simulink model "mrefrobotarm_modified_previous_y_previous_u_previous_ref_cover"  (R2018b)
settings: Solver=FixedStepAuto  StartTime=0.0  StopTime=20  RelTol=1e-3  AbsTol=1e-6
undefined symbols (not defined in the file or in its folder): cc, options
libraries: neural x396, simulink x1
(part 5 of 15)

== system mrefrobotarm_modified_previous_y_previous_u_previous_ref_cover/Feed-Forward Neural Network1/Layer 3/Delays 1 ==
  "p{3}" : Inport  PortDimensions=30
      mask Display: e = 0.06;c1 = [120 230 180]/255;c2 = ([120 230 180]+0)/(256+128);c3 = ([120 230 180]+128)/(256+128);patch([0 1 1 0],[0 0 1 1],c1);patch([0 1 1 1-e 1-e 0+e],[0 0 1 1-e 0+e 0+e],c2);patch([0 0 1 1-e 0+e 0+e],[0 1 1 1-e 1-e 0+e],c3);plot([0 1 1 0 0],[0 0 1 1 0]);
  mux : Mux  Inputs=1
      mask Display: e = 0.06;c1 = [120 150 230]/255;c2 = ([120 150 230]+0)/383;c3 = ([120 150 230]+128)/383;patch([0 1 1 0],[0 0 1 1],c1);patch([0 1 1 1-e 1-e 0+e],[0 0 1 1-e 0+e 0+e],c2);patch([0 0 1 1-e 0+e 0+e],[0 1 1 1-e 1-e 0+e],c3);plot([0 1 1 0 0],[0 0 1 1 0]);disp('Mux')
  "pd{3,2}" : Outport
      mask Display: e = 0.06;c1 = [120 230 180]/255;c2 = ([120 230 180]+0)/(256+128);c3 = ([120 230 180]+128)/(256+128);patch([0 1 1 0],[0 0 1 1],c1);patch([0 1 1 1-e 1-e 0+e],[0 0 1 1-e 0+e 0+e],c2);patch([0 0 1 1-e 0+e 0+e],[0 1 1 1-e 1-e 0+e],c3);plot([0 1 1 0 0],[0 0 1 1 0]);
  wires:
  "p{3}"/1 -> mux/1
  mux/1 -> "pd{3,2}"/1

== system mrefrobotarm_modified_previous_y_previous_u_previous_ref_cover/Feed-Forward Neural Network1/Layer 3/LW{3,2} ==
  "ad{3,2}" : Inport  PortDimensions=30
      mask Display: e = 0.06;c1 = [120 230 180]/255;c2 = ([120 230 180]+0)/(256+128);c3 = ([120 230 180]+128)/(256+128);patch([0 1 1 0],[0 0 1 1],c1);patch([0 1 1 1-e 1-e 0+e],[0 0 1 1-e 0+e 0+e],c2);patch([0 0 1 1-e 0+e 0+e],[0 1 1 1-e 1-e 0+e],c3);plot([0 1 1 0 0],[0 0 1 1 0]);
  "IW{3,2}(1,:)'" : Constant  Value=[0.245566465926212396109207247718586586415767669677734375;-0.56322081322037842454619749332778155803680419921875;-0.28991010367060410235495737651945091784000396728515625;0.3869683333504421174353637979947961866855621337890625;0.496517765752567064030387200546101666986942291259765625;-0.320943780837954883988771825897856615483760833740234375;0.0286370319336148211608605862465992686338722705841064453125;-0.15395906619913668489374458658858202397823333740234375;0.51493301451079076525019218024681322276592254638671875;-0.026941881639260277514491548345176852308213710784912109375;-0.05589778476223307424053388103857287205755710601806640625;0.1600136141061642980343293629630352370440959930419921875;-0.2212967731759021561277478440388222225010395050048828125;-0.168090459815553538991395043922238983213901519775390625;-0.4615503546136172641212169764912687242031097412109375;-0.60839853859597503582534727684105746448040008544921875;0.1504483327033876438605375369661487638950347900390625;-0.4073407234202310878146136019495315849781036376953125;0.331316055045982882365507293798145838081836700439453125;-0.1747391852843100945591459094430319964885711669921875;-0.19591165143500910428286942988052032887935638427734375;0.1816474984983245388736605718804639764130115509033203125;0.3783772749804861224021124144201166927814483642578125;0.046857186277910960192638611943038995377719402313232421875;-0.292883801455053660589555875048972666263580322265625;0.480373124807368323541112431485089473426342010498046875;-0.0158594532240923617727457184400918777100741863250732421875;-0.0228072195102398851684899483416302246041595935821533203125;-0.55934110245892210144802447757683694362640380859375;0.2422309302660256846717601320051471702754497528076171875]
      mask Display: e = 0.06;c1 = [120 150 230]/255;c2 = ([120 150 230]+0)/383;c3 = ([120 150 230]+128)/383;patch([0 1 1 0],[0 0 1 1],c1);patch([0 1 1 1-e 1-e 0+e],[0 0 1 1-e 0+e 0+e],c2);patch([0 0 1 1-e 0+e 0+e],[0 1 1 1-e 1-e 0+e],c3);plot([0 1 1 0 0],[0 0 1 1 0]);disp('weights');
  Mux : Mux  Inputs=1
      mask Display: e = 0.06;c1 = [120 150 230]/255;c2 = ([120 150 230]+0)/383;c3 = ([120 150 230]+128)/383;patch([0 1 1 0],[0 0 1 1],c1);patch([0 1 1 1-e 1-e 0+e],[0 0 1 1-e 0+e 0+e],c2);patch([0 0 1 1-e 0+e 0+e],[0 1 1 1-e 1-e 0+e],c3);plot([0 1 1 0 0],[0 0 1 1 0]);disp('Mux');
  dotprod1 : neural/Weight Functions/dotprod
  "lz{3,2}" : Outport
      mask Display: e = 0.06;c1 = [120 230 180]/255;c2 = ([120 230 180]+0)/(256+128);c3 = ([120 230 180]+128)/(256+128);patch([0 1 1 0],[0 0 1 1],c1);patch([0 1 1 1-e 1-e 0+e],[0 0 1 1-e 0+e 0+e],c2);patch([0 0 1 1-e 0+e 0+e],[0 1 1 1-e 1-e 0+e],c3);plot([0 1 1 0 0],[0 0 1 1 0]);
  wires:
  "IW{3,2}(1,:)'"/1 -> dotprod1/1
  "ad{3,2}"/1 -> dotprod1/2
  dotprod1/1 -> Mux/1
  Mux/1 -> "lz{3,2}"/1

== system mrefrobotarm_modified_previous_y_previous_u_previous_ref_cover/cov_error/Layer 1/Delays 1 ==
  "p{1}" : Inport  PortDimensions=10
      mask Display: e = 0.06;c1 = [120 230 180]/255;c2 = ([120 230 180]+0)/(256+128);c3 = ([120 230 180]+128)/(256+128);patch([0 1 1 0],[0 0 1 1],c1);patch([0 1 1 1-e 1-e 0+e],[0 0 1 1-e 0+e 0+e],c2);patch([0 0 1 1-e 0+e 0+e],[0 1 1 1-e 1-e 0+e],c3);plot([0 1 1 0 0],[0 0 1 1 0]);
  mux : Mux  Inputs=1
      mask Display: e = 0.06;c1 = [120 150 230]/255;c2 = ([120 150 230]+0)/383;c3 = ([120 150 230]+128)/383;patch([0 1 1 0],[0 0 1 1],c1);patch([0 1 1 1-e 1-e 0+e],[0 0 1 1-e 0+e 0+e],c2);patch([0 0 1 1-e 0+e 0+e],[0 1 1 1-e 1-e 0+e],c3);plot([0 1 1 0 0],[0 0 1 1 0]);disp('Mux')
  "pd{1,1}" : Outport
      mask Display: e = 0.06;c1 = [120 230 180]/255;c2 = ([120 230 180]+0)/(256+128);c3 = ([120 230 180]+128)/(256+128);patch([0 1 1 0],[0 0 1 1],c1);patch([0 1 1 1-e 1-e 0+e],[0 0 1 1-e 0+e 0+e],c2);patch([0 0 1 1-e 0+e 0+e],[0 1 1 1-e 1-e 0+e],c3);plot([0 1 1 0 0],[0 0 1 1 0]);
  wires:
  "p{1}"/1 -> mux/1
  mux/1 -> "pd{1,1}"/1

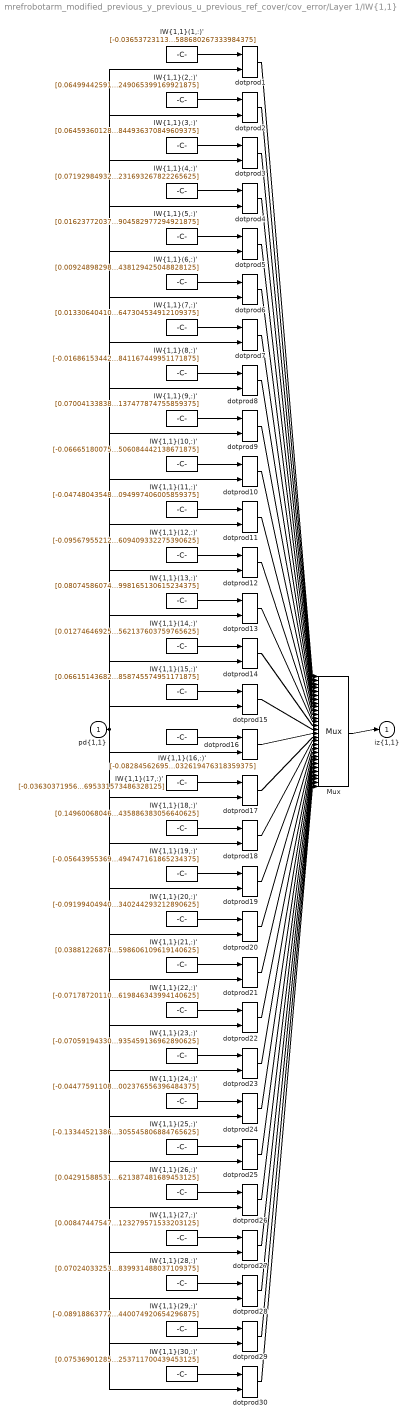
== system mrefrobotarm_modified_previous_y_previous_u_previous_ref_cover/cov_error/Layer 1/IW{1,1} ==
  "pd{1,1}" : Inport  PortDimensions=10
      mask Display: e = 0.06;c1 = [120 230 180]/255;c2 = ([120 230 180]+0)/(256+128);c3 = ([120 230 180]+128)/(256+128);patch([0 1 1 0],[0 0 1 1],c1);patch([0 1 1 1-e 1-e 0+e],[0 0 1 1-e 0+e 0+e],c2);patch([0 0 1 1-e 0+e 0+e],[0 1 1 1-e 1-e 0+e],c3);plot([0 1 1 0 0],[0 0 1 1 0]);
  "IW{1,1}(1,:)'" : Constant  Value=[-0.03653723113104710706888766935662715695798397064208984375;0.038360550813672546210941760591595084406435489654541015625;0.000744509118963375903475776507178807150921784341335296630859375;0.01020321352110764752396665500100425560958683490753173828125;0.03184344501089390877535123536290484480559825897216796875;-0.0104486251976073467317984722058099578134715557098388671875;0.0202694443671842493281953778705428703688085079193115234375;0.0134132205307559322637889209772765752859413623809814453125;0.005389856573634030194319688433779447223059833049774169921875;-0.0149595228110809795596392035577082424424588680267333984375]
      mask Display: e = 0.06;c1 = [120 150 230]/255;c2 = ([120 150 230]+0)/383;c3 = ([120 150 230]+128)/383;patch([0 1 1 0],[0 0 1 1],c1);patch([0 1 1 1-e 1-e 0+e],[0 0 1 1-e 0+e 0+e],c2);patch([0 0 1 1-e 0+e 0+e],[0 1 1 1-e 1-e 0+e],c3);plot([0 1 1 0 0],[0 0 1 1 0]);disp('Weights');
  "IW{1,1}(10,:)'" : Constant  Value=[-0.06665180075754757738071276662594755180180072784423828125;0.1725890573163153252078672039715456776320934295654296875;-0.11087739901806976938747340000190888531506061553955078125;0.0024050791294655017582559963784660794772207736968994140625;0.1336375942462473265237576924846507608890533447265625;-0.2164844012016073626636369908737833611667156219482421875;0.08265398868573266277781641520050470717251300811767578125;0.0199606436467924842903531867932542809285223484039306640625;-0.06163090580996570533311995632175239734351634979248046875;-0.1325037227429546049517483652380178682506084442138671875]
      mask Display: e = 0.06;c1 = [120 150 230]/255;c2 = ([120 150 230]+0)/383;c3 = ([120 150 230]+128)/383;patch([0 1 1 0],[0 0 1 1],c1);patch([0 1 1 1-e 1-e 0+e],[0 0 1 1-e 0+e 0+e],c2);patch([0 0 1 1-e 0+e 0+e],[0 1 1 1-e 1-e 0+e],c3);plot([0 1 1 0 0],[0 0 1 1 0]);disp('Weights');
  "IW{1,1}(11,:)'" : Constant  Value=[-0.047480435485290108099665218333029770292341709136962890625;0.0177663753596795093159244061098434031009674072265625;-0.008859429055046309786636271610404946841299533843994140625;-9.353262095238953541774529210073296781047247350215911865234375e-05;0.00863141728509585724748998103450503549538552761077880859375;-0.017571241636531724494840744910106877796351909637451171875;0.0172601667045389449428594019764204858802258968353271484375;0.01290902980637330908775251003817174932919442653656005859375;-0.01394180518576602911817730046095675788819789886474609375;-0.0146746017718865327805755072176907560788094997406005859375]
      mask Display: e = 0.06;c1 = [120 150 230]/255;c2 = ([120 150 230]+0)/383;c3 = ([120 150 230]+128)/383;patch([0 1 1 0],[0 0 1 1],c1);patch([0 1 1 1-e 1-e 0+e],[0 0 1 1-e 0+e 0+e],c2);patch([0 0 1 1-e 0+e 0+e],[0 1 1 1-e 1-e 0+e],c3);plot([0 1 1 0 0],[0 0 1 1 0]);disp('Weights');
  "IW{1,1}(12,:)'" : Constant  Value=[-0.09567955212930388808612036655176780186593532562255859375;0.143091552287510637153644665886531583964824676513671875;-0.05922321993797903527667614298479747958481311798095703125;-0.006667507299044243829211353613573010079562664031982421875;0.0723254104182122770083651630557142198085784912109375;-0.14388483840147181513913210437749512493610382080078125;0.06501747925671878813869142277326318435370922088623046875;-0.006383587513423642605114860515413965913467109203338623046875;0.004152052272585834806484239578594497288577258586883544921875;-0.08406215735264589705710847056252532638609409332275390625]
      mask Display: e = 0.06;c1 = [120 150 230]/255;c2 = ([120 150 230]+0)/383;c3 = ([120 150 230]+128)/383;patch([0 1 1 0],[0 0 1 1],c1);patch([0 1 1 1-e 1-e 0+e],[0 0 1 1-e 0+e 0+e],c2);patch([0 0 1 1-e 0+e 0+e],[0 1 1 1-e 1-e 0+e],c3);plot([0 1 1 0 0],[0 0 1 1 0]);disp('Weights');
  "IW{1,1}(13,:)'" : Constant  Value=[0.080745860743808572923541078125708736479282379150390625;-0.12247829723255272693638318060038727708160877227783203125;0.043165689290379748166426310262977494858205318450927734375;0.003932714165185059555784885532148109632544219493865966796875;-0.055278300630651810987359340288094244897365570068359375;0.108111091007423942844667408280656673014163970947265625;-0.04282653182589897522536404039783519692718982696533203125;-0.000158017013399111669498531274058450435404665768146514892578125;-0.007567255393071993518905316022937768138945102691650390625;0.057496818548176308050212668376843794248998165130615234375]
      mask Display: e = 0.06;c1 = [120 150 230]/255;c2 = ([120 150 230]+0)/383;c3 = ([120 150 230]+128)/383;patch([0 1 1 0],[0 0 1 1],c1);patch([0 1 1 1-e 1-e 0+e],[0 0 1 1-e 0+e 0+e],c2);patch([0 0 1 1-e 0+e 0+e],[0 1 1 1-e 1-e 0+e],c3);plot([0 1 1 0 0],[0 0 1 1 0]);disp('Weights');
  "IW{1,1}(14,:)'" : Constant  Value=[0.012746469254395119408140857331090955995023250579833984375;0.000550768758065268092781463504792327512404881417751312255859375;0.003799526543546447553134637331595513387583196163177490234375;0.003055089508862786525089649813935466227121651172637939453125;-0.00144965741984122019510305978684527872246690094470977783203125;0.002199738363622001126318483699151329346932470798492431640625;-0.0039699032814268613023056531119436840526759624481201171875;-0.0033978119365018592812344166986804339103400707244873046875;0.0039464103778455612847597677728117560036480426788330078125;0.0021944975543215596881785334204550963477231562137603759765625]
      mask Display: e = 0.06;c1 = [120 150 230]/255;c2 = ([120 150 230]+0)/383;c3 = ([120 150 230]+128)/383;patch([0 1 1 0],[0 0 1 1],c1);patch([0 1 1 1-e 1-e 0+e],[0 0 1 1-e 0+e 0+e],c2);patch([0 0 1 1-e 0+e 0+e],[0 1 1 1-e 1-e 0+e],c3);plot([0 1 1 0 0],[0 0 1 1 0]);disp('Weights');
  "IW{1,1}(15,:)'" : Constant  Value=[0.06615143682911950318015215088962577283382415771484375;-0.09807285871126068810266218633842072449624538421630859375;0.04005785156533210600304784065883723087608814239501953125;0.000770935471628085154834064685047678722185082733631134033203125;-0.0649066274946534516043783469285699538886547088623046875;0.08354586220903519044878038357637706212699413299560546875;-0.0259433357333076763939772035882924683392047882080078125;0.002361324770158467097058707651058284682221710681915283203125;-0.00549328087635512184172537075710351928137242794036865234375;0.056921378046203500999933311277345637790858745574951171875]
      mask Display: e = 0.06;c1 = [120 150 230]/255;c2 = ([120 150 230]+0)/383;c3 = ([120 150 230]+128)/383;patch([0 1 1 0],[0 0 1 1],c1);patch([0 1 1 1-e 1-e 0+e],[0 0 1 1-e 0+e 0+e],c2);patch([0 0 1 1-e 0+e 0+e],[0 1 1 1-e 1-e 0+e],c3);plot([0 1 1 0 0],[0 0 1 1 0]);disp('Weights');
  "IW{1,1}(16,:)'" : Constant  Value=[-0.0828456269515249477120022447707015089690685272216796875;0.169679571756264524484691946781822480261325836181640625;-0.029594216058350338027782555627709371037781238555908203125;-0.058674232955252612897734110219971626065671443939208984375;0.10046655236704733760166874390051816590130329132080078125;-0.13381216446317178991876062355004251003265380859375;0.0861001318806440263387003142270259559154510498046875;-0.049264430999797388655014884761840221472084522247314453125;-0.01182537442875567813838078023991329246200621128082275390625;-0.0874476586597564276015503992312005721032619476318359375]
      mask Display: e = 0.06;c1 = [120 150 230]/255;c2 = ([120 150 230]+0)/383;c3 = ([120 150 230]+128)/383;patch([0 1 1 0],[0 0 1 1],c1);patch([0 1 1 1-e 1-e 0+e],[0 0 1 1-e 0+e 0+e],c2);patch([0 0 1 1-e 0+e 0+e],[0 1 1 1-e 1-e 0+e],c3);plot([0 1 1 0 0],[0 0 1 1 0]);disp('Weights');
  "IW{1,1}(17,:)'" : Constant  Value=[-0.03630371956660756460610883777917479164898395538330078125;0.044516260714754264660175664403141126967966556549072265625;-0.0192261442226275593159190435699201771058142185211181640625;0.00904620160095585303106080488078077905811369419097900390625;0.0245830690072786732514042995489944587461650371551513671875;-0.0710130650831028720215698513129609636962413787841796875;0.00812266228516002851411936802605850971303880214691162109375;-0.00868490837055533627941716900977553450502455234527587890625;-0.0145788123988003504027943790788413025438785552978515625;-0.03115176029818873815191437870453228242695331573486328125]
      mask Display: e = 0.06;c1 = [120 150 230]/255;c2 = ([120 150 230]+0)/383;c3 = ([120 150 230]+128)/383;patch([0 1 1 0],[0 0 1 1],c1);patch([0 1 1 1-e 1-e 0+e],[0 0 1 1-e 0+e 0+e],c2);patch([0 0 1 1-e 0+e 0+e],[0 1 1 1-e 1-e 0+e],c3);plot([0 1 1 0 0],[0 0 1 1 0]);disp('Weights');
  "IW{1,1}(18,:)'" : Constant  Value=[0.14960068046303398592300482050632126629352569580078125;-0.16194336111059304261772240352001972496509552001953125;0.058762005273295059293303665981511585414409637451171875;-0.00387007609215116003820167378535188618116080760955810546875;0.09454389804520513251873126137070357799530029296875;0.188653312593725142054523757906281389296054840087890625;-0.0877472860665167997407110078711411915719509124755859375;-0.07404742272622104326540437568837660364806652069091796875;-0.0174072195951593018670155998961490695364773273468017578125;0.058276842395464469037680288465708144940435886383056640625]
      mask Display: e = 0.06;c1 = [120 150 230]/255;c2 = ([120 150 230]+0)/383;c3 = ([120 150 230]+128)/383;patch([0 1 1 0],[0 0 1 1],c1);patch([0 1 1 1-e 1-e 0+e],[0 0 1 1-e 0+e 0+e],c2);patch([0 0 1 1-e 0+e 0+e],[0 1 1 1-e 1-e 0+e],c3);plot([0 1 1 0 0],[0 0 1 1 0]);disp('Weights');
  "IW{1,1}(19,:)'" : Constant  Value=[-0.056439553699023682631352727412377134896814823150634765625;0.1361506813480790611947668367065489292144775390625;-0.07616655116593258612045502786713768728077411651611328125;0.00587875707181872986240023237769491970539093017578125;0.058816112037137734114278231345451786182820796966552734375;-0.14498305620830598261505883783684112131595611572265625;0.0722337159921333793466402539706905372440814971923828125;0.007809434842050935569879310804708438809029757976531982421875;0.00627591618905247623783072441483454895205795764923095703125;-0.0931938535617256869070246239061816595494747161865234375]
      mask Display: e = 0.06;c1 = [120 150 230]/255;c2 = ([120 150 230]+0)/383;c3 = ([120 150 230]+128)/383;patch([0 1 1 0],[0 0 1 1],c1);patch([0 1 1 1-e 1-e 0+e],[0 0 1 1-e 0+e 0+e],c2);patch([0 0 1 1-e 0+e 0+e],[0 1 1 1-e 1-e 0+e],c3);plot([0 1 1 0 0],[0 0 1 1 0]);disp('Weights');
  "IW{1,1}(2,:)'" : Constant  Value=[0.064994425912171693848762288325815461575984954833984375;-0.0918874697437537524269401956189540214836597442626953125;0.03093606243520696796878155510057695209980010986328125;-6.907580963489280516387491815066823619417846202850341796875e-05;-0.059612760305134189497966445969723281450569629669189453125;0.074026469344271095263110282758134417235851287841796875;-0.03357215078970469945840449099705438129603862762451171875;-0.00014466226318381333014462253316878559417091310024261474609375;-0.002966189554747650745925025006499708979390561580657958984375;0.05391906230681069167598451485901023261249065399169921875]
      mask Display: e = 0.06;c1 = [120 150 230]/255;c2 = ([120 150 230]+0)/383;c3 = ([120 150 230]+128)/383;patch([0 1 1 0],[0 0 1 1],c1);patch([0 1 1 1-e 1-e 0+e],[0 0 1 1-e 0+e 0+e],c2);patch([0 0 1 1-e 0+e 0+e],[0 1 1 1-e 1-e 0+e],c3);plot([0 1 1 0 0],[0 0 1 1 0]);disp('Weights');
  "IW{1,1}(20,:)'" : Constant  Value=[-0.0919940494054823643121920895282528363168239593505859375;0.2113317007550328252563076603109948337078094482421875;-0.0945720491508910410249910682978224940598011016845703125;-0.00512048429726825841956650009478835272602736949920654296875;0.1381914866141488451578567264732555486261844635009765625;-0.2300633871765608573500827560565085150301456451416015625;0.095575735295521990764200381818227469921112060546875;0.0080174053609905447659311761299250065349042415618896484375;-0.1021830883615167107070220708919805474579334259033203125;-0.1771926836196399401845980037251138128340244293212890625]
      mask Display: e = 0.06;c1 = [120 150 230]/255;c2 = ([120 150 230]+0)/383;c3 = ([120 150 230]+128)/383;patch([0 1 1 0],[0 0 1 1],c1);patch([0 1 1 1-e 1-e 0+e],[0 0 1 1-e 0+e 0+e],c2);patch([0 0 1 1-e 0+e 0+e],[0 1 1 1-e 1-e 0+e],c3);plot([0 1 1 0 0],[0 0 1 1 0]);disp('Weights');
  "IW{1,1}(21,:)'" : Constant  Value=[0.038812268789324255724437762182787992060184478759765625;-0.04480456188123345395712959771117311902344226837158203125;0.016246819742007902187541645844248705543577671051025390625;-0.006604456541362642950365735572404446429572999477386474609375;-0.04322617002172358946499031162602477706968784332275390625;0.036167707590489532598621025272223050706088542938232421875;-0.0213454025428620706994475852980031049810349941253662109375;-0.01066227332560157510521481327714354847557842731475830078125;0.0220903568044329666475444895468172035180032253265380859375;0.034015232973375809921723345041755237616598606109619140625]
      mask Display: e = 0.06;c1 = [120 150 230]/255;c2 = ([120 150 230]+0)/383;c3 = ([120 150 230]+128)/383;patch([0 1 1 0],[0 0 1 1],c1);patch([0 1 1 1-e 1-e 0+e],[0 0 1 1-e 0+e 0+e],c2);patch([0 0 1 1-e 0+e 0+e],[0 1 1 1-e 1-e 0+e],c3);plot([0 1 1 0 0],[0 0 1 1 0]);disp('Weights');
  "IW{1,1}(22,:)'" : Constant  Value=[-0.071787201101108533141115231046569533646106719970703125;0.07820574401857889601519246980387833900749683380126953125;-0.0205035945787483790681005046963036875240504741668701171875;0.000162757991755136592441910448059161353739909827709197998046875;0.03267040847848433349209784637423581443727016448974609375;-0.06390039326101361327747696350343176163733005523681640625;0.033920185035053403155291817938632448203861713409423828125;0.0090282133815502811635678170887331361882388591766357421875;-0.0028829879164051735833396161723385375807993113994598388671875;-0.03585056750200765751657172586419619619846343994140625]
      mask Display: e = 0.06;c1 = [120 150 230]/255;c2 = ([120 150 230]+0)/383;c3 = ([120 150 230]+128)/383;patch([0 1 1 0],[0 0 1 1],c1);patch([0 1 1 1-e 1-e 0+e],[0 0 1 1-e 0+e 0+e],c2);patch([0 0 1 1-e 0+e 0+e],[0 1 1 1-e 1-e 0+e],c3);plot([0 1 1 0 0],[0 0 1 1 0]);disp('Weights');
  "IW{1,1}(23,:)'" : Constant  Value=[-0.0705919433061602819012847476187744177877902984619140625;0.0851730983976952682468208877253346145153045654296875;-0.022692421962937088519840500566715491004288196563720703125;0.0111685758662134204666216419354896061122417449951171875;0.032806928121286445254600749876772169955074787139892578125;-0.06742074813825758849983316167708835564553737640380859375;0.0328535157759104468055966208339668810367584228515625;0.01053453253065129470444905024351101019419729709625244140625;0.01012897878361995913920612366609930177219212055206298828125;-0.039103781593332477550806203225874924100935459136962890625]
      mask Display: e = 0.06;c1 = [120 150 230]/255;c2 = ([120 150 230]+0)/383;c3 = ([120 150 230]+128)/383;patch([0 1 1 0],[0 0 1 1],c1);patch([0 1 1 1-e 1-e 0+e],[0 0 1 1-e 0+e 0+e],c2);patch([0 0 1 1-e 0+e 0+e],[0 1 1 1-e 1-e 0+e],c3);plot([0 1 1 0 0],[0 0 1 1 0]);disp('Weights');
  "IW{1,1}(24,:)'" : Constant  Value=[-0.0447759110827454787084889176185242831707000732421875;0.004131345695153754681017144179122624336741864681243896484375;-0.0062302807214579536410070659258053638041019439697265625;-0.00796367441263994522981928270155549398623406887054443359375;0.005829833971947927066803440965259142103604972362518310546875;-0.004573005914818015389677885451646943693049252033233642578125;0.0141882895224129980393801275795340188778936862945556640625;0.0156532704924001730972804580233059823513031005859375;-0.0083191710719612045610293904474019655026495456695556640625;-0.000841981859197891979729178046909510158002376556396484375]
      mask Display: e = 0.06;c1 = [120 150 230]/255;c2 = ([120 150 230]+0)/383;c3 = ([120 150 230]+128)/383;patch([0 1 1 0],[0 0 1 1],c1);patch([0 1 1 1-e 1-e 0+e],[0 0 1 1-e 0+e 0+e],c2);patch([0 0 1 1-e 0+e 0+e],[0 1 1 1-e 1-e 0+e],c3);plot([0 1 1 0 0],[0 0 1 1 0]);disp('Weights');
  "IW{1,1}(25,:)'" : Constant  Value=[-0.133445213863365996775911526128766126930713653564453125;0.2078040962087924492518453689626767300069332122802734375;-0.07605030694922267076041322297896840609610080718994140625;0.015783096326577768231391729614188079722225666046142578125;0.060891000296897486443459257543509011156857013702392578125;-0.227497227035688587282180606052861548960208892822265625;0.0702492649448114292454192764125764369964599609375;0.004649515161143302592605675016557142953388392925262451171875;-0.0277183478571610512897205325089089456014335155487060546875;-0.10941849309645447496652792551685706712305545806884765625]
      mask Display: e = 0.06;c1 = [120 150 230]/255;c2 = ([120 150 230]+0)/383;c3 = ([120 150 230]+128)/383;patch([0 1 1 0],[0 0 1 1],c1);patch([0 1 1 1-e 1-e 0+e],[0 0 1 1-e 0+e 0+e],c2);patch([0 0 1 1-e 0+e 0+e],[0 1 1 1-e 1-e 0+e],c3);plot([0 1 1 0 0],[0 0 1 1 0]);disp('Weights');
  "IW{1,1}(26,:)'" : Constant  Value=[0.0429158853145547303231666091960505582392215728759765625;-0.1623163302774468796929596692280028946697711944580078125;0.1164647856859561680931136606886866502463817596435546875;-0.006527538107474729900392418358023860491812229156494140625;-0.2295472997845038054531840998606639914214611053466796875;0.2422737721148322531661278844694606959819793701171875;-0.12030037627731766936012292035229620523750782012939453125;0.0784824726129946526054226296764682047069072723388671875;0.040075783731325198555595079596969299018383026123046875;0.1698280566241636979629703319005784578621387481689453125]
      mask Display: e = 0.06;c1 = [120 150 230]/255;c2 = ([120 150 230]+0)/383;c3 = ([120 150 230]+128)/383;patch([0 1 1 0],[0 0 1 1],c1);patch([0 1 1 1-e 1-e 0+e],[0 0 1 1-e 0+e 0+e],c2);patch([0 0 1 1-e 0+e 0+e],[0 1 1 1-e 1-e 0+e],c3);plot([0 1 1 0 0],[0 0 1 1 0]);disp('Weights');
  "IW{1,1}(27,:)'" : Constant  Value=[0.008474475476937561035928325736676924861967563629150390625;0.004798968672440472038598358039962477050721645355224609375;0.004798897135086619726573875510666766786016523838043212890625;0.003963956589695572137188595007728508790023624897003173828125;0.0023822215363806264511181698395603234530426561832427978515625;0.0036413197587943659482012659367455853498540818691253662109375;-0.0007320197897932091170292157045196290710009634494781494140625;-0.00158129241006373100209003723648493178188800811767578125;0.00645894761764856557839653561359227751381695270538330078125;0.000561998278485313228387820760900694949668832123279571533203125]
      mask Display: e = 0.06;c1 = [120 150 230]/255;c2 = ([120 150 230]+0)/383;c3 = ([120 150 230]+128)/383;patch([0 1 1 0],[0 0 1 1],c1);patch([0 1 1 1-e 1-e 0+e],[0 0 1 1-e 0+e 0+e],c2);patch([0 0 1 1-e 0+e 0+e],[0 1 1 1-e 1-e 0+e],c3);plot([0 1 1 0 0],[0 0 1 1 0]);disp('Weights');
  "IW{1,1}(28,:)'" : Constant  Value=[0.0702403325348168461328413059163722209632396697998046875;-0.092832058691033392250346878427080810070037841796875;0.030669406418969154259901443992930580861866474151611328125;0.00049860917313159880230599707573446721653454005718231201171875;-0.051461616254597837560869066919622127898037433624267578125;0.07410498594144467043864921151907765306532382965087890625;-0.0274957514130889264791779424967899103648960590362548828125;0.001033874348456445720068064275665165041573345661163330078125;-0.0088852280370854373747757648516198969446122646331787109375;0.050330289296195339365791454611098743043839931488037109375]
      mask Display: e = 0.06;c1 = [120 150 230]/255;c2 = ([120 150 230]+0)/383;c3 = ([120 150 230]+128)/383;patch([0 1 1 0],[0 0 1 1],c1);patch([0 1 1 1-e 1-e 0+e],[0 0 1 1-e 0+e 0+e],c2);patch([0 0 1 1-e 0+e 0+e],[0 1 1 1-e 1-e 0+e],c3);plot([0 1 1 0 0],[0 0 1 1 0]);disp('Weights');
  "IW{1,1}(29,:)'" : Constant  Value=[-0.08918863772935513301032273147939122281968593597412109375;-0.0222917228558486245348913001862456439994275569915771484375;0.011493299695143795180474199923992273397743701934814453125;0.017864070585899123611017813573198509402573108673095703125;0.00158606683832126517906535578816829001880250871181488037109375;-0.018771650897375258271182474345550872385501861572265625;0.04637384383512467567189929695814498700201511383056640625;0.04659991018732785594824719055395689792931079864501953125;-0.056452103268618346321172651869346736930310726165771484375;0.00050464854237953766895319329677249697851948440074920654296875]
      mask Display: e = 0.06;c1 = [120 150 230]/255;c2 = ([120 150 230]+0)/383;c3 = ([120 150 230]+128)/383;patch([0 1 1 0],[0 0 1 1],c1);patch([0 1 1 1-e 1-e 0+e],[0 0 1 1-e 0+e 0+e],c2);patch([0 0 1 1-e 0+e 0+e],[0 1 1 1-e 1-e 0+e],c3);plot([0 1 1 0 0],[0 0 1 1 0]);disp('Weights');
  "IW{1,1}(3,:)'" : Constant  Value=[0.06459360128309710180616320940316654741764068603515625;-0.1098008829576446465647876493676449172198772430419921875;0.039343522245274049897734158776074764318764209747314453125;0.000339475034880201589730652766974117184872739017009735107421875;-0.0677655329999866384849127598499762825667858123779296875;0.09692833493347015327845639376391773112118244171142578125;-0.040788262438762913630885265092729241587221622467041015625;0.009020214636157243559555496403845609165728092193603515625;0.00929823323973506983552983484742071595974266529083251953125;0.06881472784452478952399445688570267520844936370849609375]
      mask Display: e = 0.06;c1 = [120 150 230]/255;c2 = ([120 150 230]+0)/383;c3 = ([120 150 230]+128)/383;patch([0 1 1 0],[0 0 1 1],c1);patch([0 1 1 1-e 1-e 0+e],[0 0 1 1-e 0+e 0+e],c2);patch([0 0 1 1-e 0+e 0+e],[0 1 1 1-e 1-e 0+e],c3);plot([0 1 1 0 0],[0 0 1 1 0]);disp('Weights');
  "IW{1,1}(30,:)'" : Constant  Value=[0.07536901285760733149032830624491907656192779541015625;-0.10320874446268528401571273889203439466655254364013671875;0.039164209840640229476349531978485174477100372314453125;0.0035176714000678386586040691241805689060129225254058837890625;-0.057445716019554893261300776430289261043071746826171875;0.08627490650482548539823568489737226627767086029052734375;-0.03131611164108465128474989569440367631614208221435546875;0.00399397273051555097567177909922975231893360614776611328125;-0.00176142644963312344948136445310638009686954319477081298828125;0.061405851531336048954035078395463642664253711700439453125]
      mask Display: e = 0.06;c1 = [120 150 230]/255;c2 = ([120 150 230]+0)/383;c3 = ([120 150 230]+128)/383;patch([0 1 1 0],[0 0 1 1],c1);patch([0 1 1 1-e 1-e 0+e],[0 0 1 1-e 0+e 0+e],c2);patch([0 0 1 1-e 0+e 0+e],[0 1 1 1-e 1-e 0+e],c3);plot([0 1 1 0 0],[0 0 1 1 0]);disp('Weights');
  "IW{1,1}(4,:)'" : Constant  Value=[0.071929849324330163984342334515531547367572784423828125;-0.0170074958380214656672446693619349389337003231048583984375;0.007071527012745660624448706954581211903132498264312744140625;-0.0059781091931944176087743159087040112353861331939697265625;-0.00859008237169353421058826114631301607005298137664794921875;0.01177138219619770255486290722046760492958128452301025390625;-0.0144827080388216893058750400768985855393111705780029296875;-0.0170175797600401780551582220368800335563719272613525390625;0.0194356523253672482109966068719586473889648914337158203125;0.01111056217860414453701967119059190736152231693267822265625]
      mask Display: e = 0.06;c1 = [120 150 230]/255;c2 = ([120 150 230]+0)/383;c3 = ([120 150 230]+128)/383;patch([0 1 1 0],[0 0 1 1],c1);patch([0 1 1 1-e 1-e 0+e],[0 0 1 1-e 0+e 0+e],c2);patch([0 0 1 1-e 0+e 0+e],[0 1 1 1-e 1-e 0+e],c3);plot([0 1 1 0 0],[0 0 1 1 0]);disp('Weights');
  "IW{1,1}(5,:)'" : Constant  Value=[0.0162377203796699835780525944528562831692397594451904296875;-0.034002509829764715476585479336790740489959716796875;0.01101302776087253847137059636906997184269130229949951171875;-0.0082731802555304594093410486266293446533381938934326171875;-0.03180611422715938496619259012732072733342647552490234375;0.0005620716167889887315833874481540988199412822723388671875;-0.0193446804195471118437144042445652303285896778106689453125;-0.0105677296506559333100216946377258864231407642364501953125;-0.000404161510742587540799541923064452930702827870845794677734375;0.0235204760678648198968243576700842822901904582977294921875]
      mask Display: e = 0.06;c1 = [120 150 230]/255;c2 = ([120 150 230]+0)/383;c3 = ([120 150 230]+128)/383;patch([0 1 1 0],[0 0 1 1],c1);patch([0 1 1 1-e 1-e 0+e],[0 0 1 1-e 0+e 0+e],c2);patch([0 0 1 1-e 0+e 0+e],[0 1 1 1-e 1-e 0+e],c3);plot([0 1 1 0 0],[0 0 1 1 0]);disp('Weights');
  "IW{1,1}(6,:)'" : Constant  Value=[0.009248982982918818596118626373936422169208526611328125;-0.00396578710273943861597256699269564705900847911834716796875;-0.0011522066167577635874275099325814153417013585567474365234375;-0.00089968250056975920987689665508924008463509380817413330078125;-0.004160404317517269780213329255502685555256903171539306640625;-0.0017712882669058392128003109888823018991388380527496337890625;-0.004165094115516804716692345067485803156159818172454833984375;-0.0035869479224276364960621865662915297434665262699127197265625;-0.00193169104661226735154821998463603449636138975620269775390625;0.00124467256381081037459879201634294076939113438129425048828125]
      mask Display: e = 0.06;c1 = [120 150 230]/255;c2 = ([120 150 230]+0)/383;c3 = ([120 150 230]+128)/383;patch([0 1 1 0],[0 0 1 1],c1);patch([0 1 1 1-e 1-e 0+e],[0 0 1 1-e 0+e 0+e],c2);patch([0 0 1 1-e 0+e 0+e],[0 1 1 1-e 1-e 0+e],c3);plot([0 1 1 0 0],[0 0 1 1 0]);disp('Weights');
  "IW{1,1}(7,:)'" : Constant  Value=[0.0133064041012517612905252661903432453982532024383544921875;-0.0988454397062259459971755859442055225372314453125;0.0302000965338972589269150859081491944380104541778564453125;-0.0307965790792437792144919939119063201360404491424560546875;-0.07809753778368000443066421212279237806797027587890625;0.042644047218570201029930188951766467653214931488037109375;-0.048764087913740199187184742868339526467025279998779296875;-0.035214794635778028097927716544290888123214244842529296875;0.046776332456605305976093944764215848408639430999755859375;0.09116110991210424341346651999629102647304534912109375]
      mask Display: e = 0.06;c1 = [120 150 230]/255;c2 = ([120 150 230]+0)/383;c3 = ([120 150 230]+128)/383;patch([0 1 1 0],[0 0 1 1],c1);patch([0 1 1 1-e 1-e 0+e],[0 0 1 1-e 0+e 0+e],c2);patch([0 0 1 1-e 0+e 0+e],[0 1 1 1-e 1-e 0+e],c3);plot([0 1 1 0 0],[0 0 1 1 0]);disp('Weights');
  "IW{1,1}(8,:)'" : Constant  Value=[-0.0168615344201069328189390716943307779729366302490234375;0.019414014113587417520445654872673912905156612396240234375;-0.000111878922707432204401711839381050594965927302837371826171875;0.00509797122548982621637048140428305487148463726043701171875;0.0141314609057716818185657103867924888618290424346923828125;-0.0060583157576709865954622813433161354623734951019287109375;0.00934523503579962229459443534551610355265438556671142578125;0.00482986475656278606283233756357731181196868419647216796875;0.0033403895069844678940296223146333431941457092761993408203125;-0.00847770218055787609656714920447484473697841167449951171875]
      mask Display: e = 0.06;c1 = [120 150 230]/255;c2 = ([120 150 230]+0)/383;c3 = ([120 150 230]+128)/383;patch([0 1 1 0],[0 0 1 1],c1);patch([0 1 1 1-e 1-e 0+e],[0 0 1 1-e 0+e 0+e],c2);patch([0 0 1 1-e 0+e 0+e],[0 1 1 1-e 1-e 0+e],c3);plot([0 1 1 0 0],[0 0 1 1 0]);disp('Weights');
  "IW{1,1}(9,:)'" : Constant  Value=[0.07004133838018537783209893632374587468802928924560546875;-0.1344853095928600084096871114525129087269306182861328125;0.050947933331309570859080082527725608088076114654541015625;-0.00547978381511436164752471000838340842165052890777587890625;-0.0654359153961116268849451671485439874231815338134765625;0.10766847066970518242978727130321203731000423431396484375;-0.05681026737331118514617855907999910414218902587890625;0.003696319744634802596794376228217515745200216770172119140625;-0.0147051471845057978027337952653397223912179470062255859375;0.07521355295656494133194058804292581044137477874755859375]
      mask Display: e = 0.06;c1 = [120 150 230]/255;c2 = ([120 150 230]+0)/383;c3 = ([120 150 230]+128)/383;patch([0 1 1 0],[0 0 1 1],c1);patch([0 1 1 1-e 1-e 0+e],[0 0 1 1-e 0+e 0+e],c2);patch([0 0 1 1-e 0+e 0+e],[0 1 1 1-e 1-e 0+e],c3);plot([0 1 1 0 0],[0 0 1 1 0]);disp('Weights');
  Mux : Mux  Inputs=30
      mask Display: e = 0.06;c1 = [120 150 230]/255;c2 = ([120 150 230]+0)/383;c3 = ([120 150 230]+128)/383;patch([0 1 1 0],[0 0 1 1],c1);patch([0 1 1 1-e 1-e 0+e],[0 0 1 1-e 0+e 0+e],c2);patch([0 0 1 1-e 0+e 0+e],[0 1 1 1-e 1-e 0+e],c3);plot([0 1 1 0 0],[0 0 1 1 0]);disp('Mux');
  dotprod{1..30} (30 alike) : neural/Weight Functions/dotprod
  "iz{1,1}" : Outport
      mask Display: e = 0.06;c1 = [120 230 180]/255;c2 = ([120 230 180]+0)/(256+128);c3 = ([120 230 180]+128)/(256+128);patch([0 1 1 0],[0 0 1 1],c1);patch([0 1 1 1-e 1-e 0+e],[0 0 1 1-e 0+e 0+e],c2);patch([0 0 1 1-e 0+e 0+e],[0 1 1 1-e 1-e 0+e],c3);plot([0 1 1 0 0],[0 0 1 1 0]);
  wires:
  "IW{1,1}(1,:)'"/1 -> dotprod1/1
  "pd{1,1}"/1 -> dotprod1/2, dotprod2/2, dotprod3/2, dotprod4/2, dotprod5/2, dotprod6/2, dotprod7/2, dotprod8/2, dotprod9/2, dotprod10/2, dotprod11/2, dotprod12/2, dotprod13/2, dotprod14/2, dotprod15/2, dotprod16/2, dotprod17/2, dotprod18/2, dotprod19/2, dotprod20/2, dotprod21/2, dotprod22/2, dotprod23/2, dotprod24/2, dotprod25/2, dotprod26/2, dotprod27/2, dotprod28/2, dotprod29/2, dotprod30/2
  dotprod1/1 -> Mux/1
  "IW{1,1}(2,:)'"/1 -> dotprod2/1
  dotprod2/1 -> Mux/2
  "IW{1,1}(3,:)'"/1 -> dotprod3/1
  dotprod3/1 -> Mux/3
  "IW{1,1}(4,:)'"/1 -> dotprod4/1
  dotprod4/1 -> Mux/4
  "IW{1,1}(5,:)'"/1 -> dotprod5/1
  dotprod5/1 -> Mux/5
  "IW{1,1}(6,:)'"/1 -> dotprod6/1
  dotprod6/1 -> Mux/6
  "IW{1,1}(7,:)'"/1 -> dotprod7/1
  dotprod7/1 -> Mux/7
  "IW{1,1}(8,:)'"/1 -> dotprod8/1
  dotprod8/1 -> Mux/8
  "IW{1,1}(9,:)'"/1 -> dotprod9/1
  dotprod9/1 -> Mux/9
  "IW{1,1}(10,:)'"/1 -> dotprod10/1
  dotprod10/1 -> Mux/10
  "IW{1,1}(11,:)'"/1 -> dotprod11/1
  dotprod11/1 -> Mux/11
  "IW{1,1}(12,:)'"/1 -> dotprod12/1
  dotprod12/1 -> Mux/12
  "IW{1,1}(13,:)'"/1 -> dotprod13/1
  dotprod13/1 -> Mux/13
  "IW{1,1}(14,:)'"/1 -> dotprod14/1
  dotprod14/1 -> Mux/14
  "IW{1,1}(15,:)'"/1 -> dotprod15/1
  dotprod15/1 -> Mux/15
  "IW{1,1}(16,:)'"/1 -> dotprod16/1
  dotprod16/1 -> Mux/16
  "IW{1,1}(17,:)'"/1 -> dotprod17/1
  dotprod17/1 -> Mux/17
  "IW{1,1}(18,:)'"/1 -> dotprod18/1
  dotprod18/1 -> Mux/18
  "IW{1,1}(19,:)'"/1 -> dotprod19/1
  dotprod19/1 -> Mux/19
  "IW{1,1}(20,:)'"/1 -> dotprod20/1
  dotprod20/1 -> Mux/20
  "IW{1,1}(21,:)'"/1 -> dotprod21/1
  dotprod21/1 -> Mux/21
  "IW{1,1}(22,:)'"/1 -> dotprod22/1
  dotprod22/1 -> Mux/22
  "IW{1,1}(23,:)'"/1 -> dotprod23/1
  dotprod23/1 -> Mux/23
  "IW{1,1}(24,:)'"/1 -> dotprod24/1
  dotprod24/1 -> Mux/24
  "IW{1,1}(25,:)'"/1 -> dotprod25/1
  dotprod25/1 -> Mux/25
  "IW{1,1}(26,:)'"/1 -> dotprod26/1
  dotprod26/1 -> Mux/26
  "IW{1,1}(27,:)'"/1 -> dotprod27/1
  dotprod27/1 -> Mux/27
  "IW{1,1}(28,:)'"/1 -> dotprod28/1
  dotprod28/1 -> Mux/28
  "IW{1,1}(29,:)'"/1 -> dotprod29/1
  dotprod29/1 -> Mux/29
  "IW{1,1}(30,:)'"/1 -> dotprod30/1
  dotprod30/1 -> Mux/30
  Mux/1 -> "iz{1,1}"/1

== system mrefrobotarm_modified_previous_y_previous_u_previous_ref_cover/cov_error/Layer 2/Delays 1 ==
  "p{2}" : Inport  PortDimensions=30
      mask Display: e = 0.06;c1 = [120 230 180]/255;c2 = ([120 230 180]+0)/(256+128);c3 = ([120 230 180]+128)/(256+128);patch([0 1 1 0],[0 0 1 1],c1);patch([0 1 1 1-e 1-e 0+e],[0 0 1 1-e 0+e 0+e],c2);patch([0 0 1 1-e 0+e 0+e],[0 1 1 1-e 1-e 0+e],c3);plot([0 1 1 0 0],[0 0 1 1 0]);
  mux : Mux  Inputs=1
      mask Display: e = 0.06;c1 = [120 150 230]/255;c2 = ([120 150 230]+0)/383;c3 = ([120 150 230]+128)/383;patch([0 1 1 0],[0 0 1 1],c1);patch([0 1 1 1-e 1-e 0+e],[0 0 1 1-e 0+e 0+e],c2);patch([0 0 1 1-e 0+e 0+e],[0 1 1 1-e 1-e 0+e],c3);plot([0 1 1 0 0],[0 0 1 1 0]);disp('Mux')
  "pd{2,1}" : Outport
      mask Display: e = 0.06;c1 = [120 230 180]/255;c2 = ([120 230 180]+0)/(256+128);c3 = ([120 230 180]+128)/(256+128);patch([0 1 1 0],[0 0 1 1],c1);patch([0 1 1 1-e 1-e 0+e],[0 0 1 1-e 0+e 0+e],c2);patch([0 0 1 1-e 0+e 0+e],[0 1 1 1-e 1-e 0+e],c3);plot([0 1 1 0 0],[0 0 1 1 0]);
  wires:
  "p{2}"/1 -> mux/1
  mux/1 -> "pd{2,1}"/1
